simulink model "CLVF"  (R2020a)
settings: Solver=FixedStepAuto  StartTime=0.0  StopTime=tsim  FixedStep=baseRate  RelTol=1e-3  EnableMultiTasking=on
undefined symbols (not defined in the file): a, a_max, a_prime, acceptableRadius, b, baseRate, BLACKMass, d, DiscIntNeverNeededParam, Discrete, drop_states_BLACK, drop_states_BLUE, drop_states_RED, F_thrusters_BLACK, F_thrusters_BLUE, F_thrusters_RED, home_states_BLACK, home_states_BLUE, home_states_RED, init_states_BLACK, init_states_BLUE, init_states_RED, k_v_rel, ka, kc, kd, Kd_tb, Kd_tblue, Kd_tr, Kd_xb, Kd_xblue, Kd_xr, Kd_yb, Kd_yblue, Kd_yr, Kp_tb, Kp_tblue, Kp_tr, Kp_xb, Kp_xblue, Kp_xr, Kp_yb, Kp_yblue, Kp_yr, noise_variance_BLACK, noise_variance_BLUE, noise_variance_RED, o_hat_B, o_hat_prime, Phase0_End, Phase1_End, Phase2_End, Phase3_End, Phase3_SubPhase1_End, Phase3_SubPhase2_End, Phase3_SubPhase3_End, Phase3_SubPhase3_End_BLACK, Phase3_SubPhase3_End_RED, Phase3_SubPhase4_End, Phase4_End ... (+18)
libraries: dspsigops x14, dspstat3 x12, raspberrypiBasiclib x10, embdlinuxlib x8, simulink x8, ctrlSharedLib x4, mspfiltlib x3, dspswit3 x2, MainLibrary x2, dsparch4 x2, sensehatlib x1
(part 3 of 8)

== system CLVF/Phase #4: Return Home/Change RED Behavior ==
  note: ARM Control Law - RED
  note: PD Control Law - RED
  note: Additional Blocks
  note: Additional blocks are stored above. Note that to control attitude using the RW, simply replace RED_Tz with RED_Tz_RW.
  note: A simple PD control law is used here to command the platform to it's initial position, as defined in the initializer.
  note: This section is reserved for any control law for the robotic manipulator.
  Action Port : ActionPort  ActionPortLabel=if(u1 == 1 | u2 == 1)
  Constant : Constant  Value=home_states_RED(3)
  Constant1 : Constant  Value=home_states_RED(1)
  Constant{2,4..6} (4 alike) : Constant  Value=0
  Constant3 : Constant  Value=home_states_RED(2)
  Custom Discrete PD (Attitude) : Subsystem
  Custom Discrete PD (X-Position) : Subsystem
  Custom Discrete PD (Y-Position) : Subsystem
  Data Store Write : DataStoreWrite  DataStoreName=RED_Tz_Shoulder
  Data Store Write1 : DataStoreWrite  DataStoreName=RED_Tz_Elbow
  Data Store Write2 : DataStoreWrite  DataStoreName=RED_Tz_Wrist
  Data Store Write3 : DataStoreWrite  DataStoreName=Float_State
  Hough Control : Subsystem
  Puck State : Constant
  RED_Fx : DataStoreWrite  DataStoreName=RED_Fx
  RED_Fy : DataStoreWrite  DataStoreName=RED_Fy
  RED_Px : DataStoreRead  DataStoreName=RED_Px
  "RED_Py " : DataStoreRead  DataStoreName=RED_Py
  RED_Rz : DataStoreRead  DataStoreName=RED_Rz
  RED_Tz : DataStoreWrite  DataStoreName=RED_Tz
  RED_Tz_RW1 : DataStoreWrite  DataStoreName=RED_Tz_RW
  Subtract : Sum  Inputs=+-
  Subtract1 : Sum  Inputs=+-
  wires:
  Constant6/1 -> Data Store Write2/1
  Constant5/1 -> Data Store Write1/1
  Constant2/1 -> RED_Tz_RW1/1
  Constant4/1 -> Data Store Write/1
  Constant1/1 -> Subtract/1
  Custom Discrete PD (Attitude)/1(Tz) -> RED_Tz/1
  Constant/1 -> Hough Control/1(Ref)
  RED_Rz/1 -> Hough Control/2(Act)
  Constant3/1 -> Subtract1/1
  Custom Discrete PD (X-Position)/1(Fx) -> RED_Fx/1
  Subtract/1 -> Custom Discrete PD (X-Position)/1(ex)
  Hough Control/1(Err) -> Custom Discrete PD (Attitude)/1(ez)
  Custom Discrete PD (Y-Position)/1(Fy) -> RED_Fy/1
  RED_Px/1 -> Subtract/2
  "RED_Py "/1 -> Subtract1/2
  Subtract1/1 -> Custom Discrete PD (Y-Position)/1(ey)
  Puck State/1 -> Data Store Write3/1

== system CLVF/Phase #4: Return Home/Is this a simulation? ==
  Constant : Constant  Value=simMode  SampleTime=-1
  isSim : Outport  VectorParamsAs1DForOutWhenUnconnected=off
  wires:
  Constant/1 -> isSim/1

== system CLVF/Phase #5: Hold Home/Change BLACK Behavior ==
  note: Additional Blocks
  note: PD Control Law - BLACK
  note: A simple PD control law is used here to command the platform to it's initial position, as defined in the initializer.
  note: Additional blocks are stored here.
  Action Port : ActionPort  ActionPortLabel=if(u1 == 2 | u2 == 1)
  BLACK_Fx : DataStoreWrite  DataStoreName=BLACK_Fx
  BLACK_Fy : DataStoreWrite  DataStoreName=BLACK_Fy
  BLACK_Px : DataStoreRead  DataStoreName=BLACK_Px
  "BLACK_Py " : DataStoreRead  DataStoreName=BLACK_Py
  BLACK_Rz : DataStoreRead  DataStoreName=BLACK_Rz
  BLACK_Tz : DataStoreWrite  DataStoreName=BLACK_Tz
  Constant : Constant  Value=home_states_BLACK(1)
  Constant2 : Constant  Value=home_states_BLACK(2)
  Constant3 : Constant  Value=home_states_BLACK(3)
  Custom Discrete PD (Attitude) : Subsystem
  Custom Discrete PD (X-Position) : Subsystem
  Custom Discrete PD (Y-Position) : Subsystem
  Data Store Write3 : DataStoreWrite  DataStoreName=Float_State
  Hough Control : Subsystem
  Puck State : Constant
  Subtract : Sum  Inputs=+-
  Subtract1 : Sum  Inputs=+-
  wires:
  Custom Discrete PD (X-Position)/1(Fx) -> BLACK_Fx/1
  "BLACK_Py "/1 -> Subtract1/2
  Subtract1/1 -> Custom Discrete PD (Y-Position)/1(ey)
  Custom Discrete PD (Y-Position)/1(Fy) -> BLACK_Fy/1
  Constant3/1 -> Hough Control/1(Ref)
  Constant/1 -> Subtract/1
  Constant2/1 -> Subtract1/1
  Subtract/1 -> Custom Discrete PD (X-Position)/1(ex)
  Hough Control/1(Err) -> Custom Discrete PD (Attitude)/1(ez)
  Custom Discrete PD (Attitude)/1(Tz) -> BLACK_Tz/1
  BLACK_Px/1 -> Subtract/2
  BLACK_Rz/1 -> Hough Control/2(Act)
  Puck State/1 -> Data Store Write3/1

== system CLVF/Phase #5: Hold Home/Change BLUE Behavior ==
  note: PD Control Law - WHITE
  note: Additional blocks are stored here.
  note: A simple PD control law is used here to command the platform to it's initial position, as defined in the initializer.
  note: Additional Blocks
  Action Port : ActionPort  ActionPortLabel=if(u1 == 3 | u2 == 1)
  BLUE_Fx : DataStoreWrite  DataStoreName=BLUE_Fx
  BLUE_Fy : DataStoreWrite  DataStoreName=BLUE_Fy
  BLUE_Px : DataStoreRead  DataStoreName=BLUE_Px
  "BLUE_Py " : DataStoreRead  DataStoreName=BLUE_Py
  BLUE_Rz : DataStoreRead  DataStoreName=BLUE_Rz
  BLUE_Tz : DataStoreWrite  DataStoreName=BLUE_Tz
  Custom Discrete PD (Attitude) : Subsystem
  Custom Discrete PD (X-Position) : Subsystem
  Custom Discrete PD (Y-Position) : Subsystem
  Data Store Write3 : DataStoreWrite  DataStoreName=Float_State
  Desired Attitude (BLUE) : Constant  Value=home_states_BLUE(3)  SampleTime=-1
  Desired Px (BLUE) : Constant  Value=home_states_BLUE(1)  SampleTime=-1
  Desired Py (BLUE) : Constant  Value=home_states_BLUE(2)  SampleTime=-1
  Hough Control : Subsystem
  Puck State : Constant
  Subtract : Sum  Inputs=+-
  Subtract1 : Sum  Inputs=+-
  wires:
  Puck State/1 -> Data Store Write3/1
  Custom Discrete PD (Y-Position)/1(Fy) -> BLUE_Fy/1
  Custom Discrete PD (X-Position)/1(Fx) -> BLUE_Fx/1
  Subtract1/1 -> Custom Discrete PD (Y-Position)/1(ey)
  "BLUE_Py "/1 -> Subtract1/2
  Desired Px (BLUE)/1 -> Subtract/1
  Hough Control/1(Err) -> Custom Discrete PD (Attitude)/1(ez)
  Subtract/1 -> Custom Discrete PD (X-Position)/1(ex)
  Custom Discrete PD (Attitude)/1(Tz) -> BLUE_Tz/1
  BLUE_Rz/1 -> Hough Control/2(Act)
  Desired Py (BLUE)/1 -> Subtract1/1
  BLUE_Px/1 -> Subtract/2
  Desired Attitude (BLUE)/1 -> Hough Control/1(Ref)

== system CLVF/Phase #5: Hold Home/Change RED Behavior ==
  note: PD Control Law - RED
  note: ARM Control Law - RED
  note: Additional Blocks
  note: Additional blocks are stored above. Note that to control attitude using the RW, simply replace RED_Tz with RED_Tz_RW.
  note: A simple PD control law is used here to command the platform to it's home position, as defined in the initializer.
  note: This section is reserved for any control law for the robotic manipulator.
  Action Port : ActionPort  ActionPortLabel=if(u1 == 1 | u2 == 1)
  Constant : Constant  Value=home_states_RED(1)
  Constant{1,4..6} (4 alike) : Constant  Value=0
  Constant2 : Constant  Value=home_states_RED(2)
  Constant3 : Constant  Value=home_states_RED(3)
  Custom Discrete PD (Attitude) : Subsystem
  Custom Discrete PD (X-Position) : Subsystem
  Custom Discrete PD (Y-Position) : Subsystem
  Data Store Write : DataStoreWrite  DataStoreName=RED_Tz_Shoulder
  Data Store Write1 : DataStoreWrite  DataStoreName=RED_Tz_Elbow
  Data Store Write2 : DataStoreWrite  DataStoreName=RED_Tz_Wrist
  Data Store Write3 : DataStoreWrite  DataStoreName=Float_State
  Hough Control : Subsystem
  Puck State : Constant
  RED_Fx : DataStoreWrite  DataStoreName=RED_Fx
  RED_Fy : DataStoreWrite  DataStoreName=RED_Fy
  RED_Px : DataStoreRead  DataStoreName=RED_Px
  "RED_Py " : DataStoreRead  DataStoreName=RED_Py
  RED_Rz : DataStoreRead  DataStoreName=RED_Rz
  RED_Tz : DataStoreWrite  DataStoreName=RED_Tz
  RED_Tz_RW : DataStoreWrite  DataStoreName=RED_Tz_RW
  Subtract : Sum  Inputs=+-
  Subtract1 : Sum  Inputs=+-
  wires:
  Constant1/1 -> RED_Tz_RW/1
  Constant5/1 -> Data Store Write1/1
  Constant4/1 -> Data Store Write/1
  Constant6/1 -> Data Store Write2/1
  "RED_Py "/1 -> Subtract1/2
  Custom Discrete PD (Attitude)/1(Tz) -> RED_Tz/1
  Subtract1/1 -> Custom Discrete PD (Y-Position)/1(ey)
  Hough Control/1(Err) -> Custom Discrete PD (Attitude)/1(ez)
  RED_Px/1 -> Subtract/2
  Custom Discrete PD (X-Position)/1(Fx) -> RED_Fx/1
  Subtract/1 -> Custom Discrete PD (X-Position)/1(ex)
  Custom Discrete PD (Y-Position)/1(Fy) -> RED_Fy/1
  Constant/1 -> Subtract/1
  Constant3/1 -> Hough Control/1(Ref)
  RED_Rz/1 -> Hough Control/2(Act)
  Constant2/1 -> Subtract1/1
  Puck State/1 -> Data Store Write3/1

== system CLVF/Phase #5: Hold Home/Is this a simulation? ==
  Constant : Constant  Value=simMode  SampleTime=-1
  isSim : Outport  VectorParamsAs1DForOutWhenUnconnected=off
  wires:
  Constant/1 -> isSim/1

== system CLVF/Phase #6: Stop Floating and Spin Down RW/Change BLACK Behavior ==
  note: At the end of the experiment, the pucks must be turned off.
  note: At the end of the experiment, all thrust and arms movement must cease.
  Action Port : ActionPort  ActionPortLabel=if(u1 == 2 | u2 == 1)
  BLACK_Fx : DataStoreWrite  DataStoreName=BLACK_Fx
  BLACK_Fy : DataStoreWrite  DataStoreName=BLACK_Fy
  BLACK_Tz : DataStoreWrite  DataStoreName=BLACK_Tz
  Constant3 : Constant  Value=0
  Constant4 : Constant  Value=0
  Constant5 : Constant  Value=0
  Data Store Write3 : DataStoreWrite  DataStoreName=Float_State
  Puck State : Constant  Value=0
  wires:
  Constant3/1 -> BLACK_Fx/1
  Constant5/1 -> BLACK_Tz/1
  Constant4/1 -> BLACK_Fy/1
  Puck State/1 -> Data Store Write3/1

== system CLVF/Phase #6: Stop Floating and Spin Down RW/Change BLUE Behavior ==
  note: Before getting good data, the platforms must NOT be floating. So, float is set to be "off".
  note: For the initialization phase, we do not want any thrust. Thus, all commanded forces are zero.
  Action Port : ActionPort  ActionPortLabel=if(u1 == 3 | u2 == 1)
  BLUE_Fx : DataStoreWrite  DataStoreName=BLUE_Fx
  BLUE_Fy : DataStoreWrite  DataStoreName=BLUE_Fy
  BLUE_Tz : DataStoreWrite  DataStoreName=BLUE_Tz
  Constant3 : Constant  Value=0
  Constant4 : Constant  Value=0
  Constant5 : Constant  Value=0
  Data Store Write4 : DataStoreWrite  DataStoreName=Float_State
  Puck State : Constant  Value=0
  wires:
  Constant3/1 -> BLUE_Fx/1
  Constant5/1 -> BLUE_Tz/1
  Constant4/1 -> BLUE_Fy/1
  Puck State/1 -> Data Store Write4/1

== system CLVF/Phase #6: Stop Floating and Spin Down RW/Change RED Behavior ==
  note: At the end of the experiment, the pucks must be turned off.
  note: At the end of the experiment, all thrust and arms movement must cease.
  note: Once the platform has settled, the RW must be slowly desaturated (assuming it has been used).
  Action Port : ActionPort  ActionPortLabel=if(u1 == 1 | u2 == 1)
  Constant{,1..2,4..6} (6 alike) : Constant  Value=0
  Data Store Write : DataStoreWrite  DataStoreName=RED_Tz_Shoulder
  Data Store Write1 : DataStoreWrite  DataStoreName=RED_Tz_Elbow
  Data Store Write2 : DataStoreWrite  DataStoreName=RED_Tz_Wrist
  Data Store Write3 : DataStoreWrite  DataStoreName=Float_State
  Gain : Gain  Gain=-1
  Puck State : Constant  Value=0
  RED_Fx : DataStoreWrite  DataStoreName=RED_Fx
  RED_Fy : DataStoreWrite  DataStoreName=RED_Fy
  RED_Tz : DataStoreWrite  DataStoreName=RED_Tz
  RED_Tz_RW : DataStoreWrite  DataStoreName=RED_Tz_RW
  RED_dRz_Speed : DataStoreRead  DataStoreName=RED_dRz_RW_Sat
  Saturation : Saturate  UpperLimit=0.005  LowerLimit=-0.005
  wires:
  Constant/1 -> RED_Fx/1
  Constant6/1 -> Data Store Write2/1
  Constant5/1 -> Data Store Write1/1
  RED_dRz_Speed/1 -> Gain/1
  Constant4/1 -> Data Store Write/1
  Saturation/1 -> RED_Tz_RW/1
  Constant1/1 -> RED_Fy/1
  Gain/1 -> Saturation/1
  Constant2/1 -> RED_Tz/1
  Puck State/1 -> Data Store Write3/1

== system CLVF/Phase #6: Stop Floating and Spin Down RW/Is this a simulation? ==
  Constant : Constant  Value=simMode  SampleTime=-1
  isSim : Outport  VectorParamsAs1DForOutWhenUnconnected=off
  wires:
  Constant/1 -> isSim/1

== system CLVF/Simulate Plant Dynamics/BLACK Dynamics Model ==
  control_inputs : Inport
  Acceleration to Velocity : DiscreteIntegrator  SampleTime=-1  ICPrevOutput=DiscIntNeverNeededParam  ICPrevScaledInput=DiscIntNeverNeededParam
  MATLAB Function : MATLAB Function  TreatAsAtomicUnit=on
  Random Number : RandomNumber  Variance=noise_variance_BLACK
  Sum : Sum  Inputs=|++
  Velocity to Position : DiscreteIntegrator  InitialCondition=drop_states_BLACK  SampleTime=-1  ICPrevOutput=DiscIntNeverNeededParam  ICPrevScaledInput=DiscIntNeverNeededParam
  states : Outport  VectorParamsAs1DForOutWhenUnconnected=off
  wires:
  control_inputs/1 -> MATLAB Function/1(control_inputs)
  MATLAB Function/1(x_ddot) -> Acceleration to Velocity/1
  Acceleration to Velocity/1 -> Velocity to Position/1
  Velocity to Position/1 -> Sum/1
  Sum/1 -> states/1
  Random Number/1 -> Sum/2

== system CLVF/Simulate Plant Dynamics/BLUE  Dynamics Model ==
  control_inputs : Inport
  Acceleration to Velocity : DiscreteIntegrator  SampleTime=-1  ICPrevOutput=DiscIntNeverNeededParam  ICPrevScaledInput=DiscIntNeverNeededParam
  MATLAB Function : MATLAB Function  TreatAsAtomicUnit=on
  Random Number : RandomNumber  Variance=noise_variance_BLUE
  Sum : Sum  Inputs=|++
  Velocity to Position : DiscreteIntegrator  InitialCondition=drop_states_BLUE  SampleTime=-1  ICPrevOutput=DiscIntNeverNeededParam  ICPrevScaledInput=DiscIntNeverNeededParam
  states : Outport  VectorParamsAs1DForOutWhenUnconnected=off
  wires:
  control_inputs/1 -> MATLAB Function/1(control_inputs)
  MATLAB Function/1(x_ddot) -> Acceleration to Velocity/1
  Acceleration to Velocity/1 -> Velocity to Position/1
  Velocity to Position/1 -> Sum/1
  Sum/1 -> states/1
  Random Number/1 -> Sum/2

== system CLVF/Simulate Plant Dynamics/RED Dynamics Model ==
  control_inputs : Inport
  Acceleration to Velocity : DiscreteIntegrator  SampleTime=-1  ICPrevOutput=DiscIntNeverNeededParam  ICPrevScaledInput=DiscIntNeverNeededParam
  MATLAB Function : MATLAB Function  TreatAsAtomicUnit=on
  Random Number : RandomNumber  Variance=noise_variance_RED
  Sum : Sum  Inputs=|++
  Velocity to Position : DiscreteIntegrator  InitialCondition=drop_states_RED  SampleTime=-1  ICPrevOutput=DiscIntNeverNeededParam  ICPrevScaledInput=DiscIntNeverNeededParam
  states : Outport  VectorParamsAs1DForOutWhenUnconnected=off
  wires:
  control_inputs/1 -> MATLAB Function/1(control_inputs)
  MATLAB Function/1(x_ddot) -> Acceleration to Velocity/1
  Acceleration to Velocity/1 -> Velocity to Position/1
  Velocity to Position/1 -> Sum/1
  Sum/1 -> states/1
  Random Number/1 -> Sum/2

== system CLVF/Simulate Plant Dynamics/Sample and Hold Data to Match PhaseSpace (BLACK) ==
  states : Inport
  Constant1 : Constant  Value=serverRate
  Data Store Read2 : DataStoreRead  DataStoreName=Univ_Time
  MATLAB Function : MATLAB Function  TreatAsAtomicUnit=on
  Sample and Hold1 : dspsigops/Sample and Hold  trig=Rising edge  initCond=drop_states_BLACK  latchinput=off
  states_hold : Outport  VectorParamsAs1DForOutWhenUnconnected=off
  wires:
  states/1 -> Sample and Hold1/1
  Data Store Read2/1 -> MATLAB Function/1(TIME)
  Constant1/1 -> MATLAB Function/2(SERVER)
  MATLAB Function/1(y) -> Sample and Hold1/Trigger
  Sample and Hold1/1 -> states_hold/1

== system CLVF/Simulate Plant Dynamics/Sample and Hold Data to Match PhaseSpace (BLUE) ==
  states : Inport
  Constant1 : Constant  Value=serverRate
  Data Store Read2 : DataStoreRead  DataStoreName=Univ_Time
  MATLAB Function : MATLAB Function  TreatAsAtomicUnit=on
  Sample and Hold1 : dspsigops/Sample and Hold  trig=Rising edge  initCond=drop_states_BLUE  latchinput=off
  states_hold : Outport  VectorParamsAs1DForOutWhenUnconnected=off
  wires:
  states/1 -> Sample and Hold1/1
  Data Store Read2/1 -> MATLAB Function/1(TIME)
  Constant1/1 -> MATLAB Function/2(SERVER)
  MATLAB Function/1(y) -> Sample and Hold1/Trigger
  Sample and Hold1/1 -> states_hold/1

== system CLVF/Simulate Plant Dynamics/Sample and Hold Data to Match PhaseSpace (RED) ==
  states : Inport
  Constant : Constant  Value=serverRate
  Data Store Read1 : DataStoreRead  DataStoreName=Univ_Time
  MATLAB Function : MATLAB Function  TreatAsAtomicUnit=on
  Sample and Hold : dspsigops/Sample and Hold  trig=Rising edge  initCond=drop_states_RED  latchinput=off
  "states_hold " : Outport  VectorParamsAs1DForOutWhenUnconnected=off
  wires:
  Data Store Read1/1 -> MATLAB Function/1(TIME)
  Constant/1 -> MATLAB Function/2(SERVER)
  MATLAB Function/1(y) -> Sample and Hold/Trigger
  Sample and Hold/1 -> "states_hold "/1
  states/1 -> Sample and Hold/1

== system CLVF/Simulate Plant Dynamics/x_dot -> x1 ==
  note: dy/dt ~= (y2-y1)/deltaT
  y(t) : Inport
  Delay1 : Delay  DelayLength=1  InitialConditionSource=Input port
      settings: InputPortMap=u0,p4
  Hold this value : Subsystem  TreatAsAtomicUnit=on
  Sum6 : Sum  Inputs=-+|
  divide by delta T : Gain  Gain=1/serverRate
  "if we went through a \"step\"" : If  IfExpression=u1 ~= 0  ShowElse=off
  dy(t)/dt : Outport  VectorParamsAs1DForOutWhenUnconnected=off
  wires:
  divide by delta T/1 -> dy(t)/dt/1
  Delay1/1 -> Sum6/1
  "if we went through a \"step\""/1 -> Hold this value/Action
  Hold this value/1(Out1) -> divide by delta T/1
  Sum6/1 -> "if we went through a \"step\""/1, Hold this value/1(In1)
  y(t)/1 -> Sum6/2, Delay1/2, Delay1/1

== system CLVF/Simulate Plant Dynamics/x_dot -> x10 ==
  note: dy/dt ~= (y2-y1)/deltaT
  y(t) : Inport
  Delay1 : Delay  DelayLength=1  InitialConditionSource=Input port
      settings: InputPortMap=u0,p4
  Hold this value : Subsystem  TreatAsAtomicUnit=on
  Sum6 : Sum  Inputs=-+|
  divide by delta T : Gain  Gain=1/serverRate
  "if we went through a \"step\"" : If  IfExpression=u1 ~= 0  ShowElse=off
  dy(t)/dt : Outport  VectorParamsAs1DForOutWhenUnconnected=off
  wires:
  divide by delta T/1 -> dy(t)/dt/1
  Delay1/1 -> Sum6/1
  "if we went through a \"step\""/1 -> Hold this value/Action
  Hold this value/1(Out1) -> divide by delta T/1
  Sum6/1 -> "if we went through a \"step\""/1, Hold this value/1(In1)
  y(t)/1 -> Sum6/2, Delay1/2, Delay1/1

== system CLVF/Simulate Plant Dynamics/x_dot -> x11 ==
  note: dy/dt ~= (y2-y1)/deltaT
  y(t) : Inport
  Delay1 : Delay  DelayLength=1  InitialConditionSource=Input port
      settings: InputPortMap=u0,p4
  Hold this value : Subsystem  TreatAsAtomicUnit=on
  Sum6 : Sum  Inputs=-+|
  divide by delta T : Gain  Gain=1/serverRate
  "if we went through a \"step\"" : If  IfExpression=u1 ~= 0  ShowElse=off
  dy(t)/dt : Outport  VectorParamsAs1DForOutWhenUnconnected=off
  wires:
  divide by delta T/1 -> dy(t)/dt/1
  Delay1/1 -> Sum6/1
  "if we went through a \"step\""/1 -> Hold this value/Action
  Hold this value/1(Out1) -> divide by delta T/1
  Sum6/1 -> "if we went through a \"step\""/1, Hold this value/1(In1)
  y(t)/1 -> Sum6/2, Delay1/2, Delay1/1

== system CLVF/Simulate Plant Dynamics/x_dot -> x13 ==
  note: dy/dt ~= (y2-y1)/deltaT
  y(t) : Inport
  Delay1 : Delay  DelayLength=1  InitialConditionSource=Input port
      settings: InputPortMap=u0,p4
  Hold this value : Subsystem  TreatAsAtomicUnit=on
  Sum6 : Sum  Inputs=-+|
  divide by delta T : Gain  Gain=1/serverRate
  "if we went through a \"step\"" : If  IfExpression=u1 ~= 0  ShowElse=off
  dy(t)/dt : Outport  VectorParamsAs1DForOutWhenUnconnected=off
  wires:
  divide by delta T/1 -> dy(t)/dt/1
  Delay1/1 -> Sum6/1
  "if we went through a \"step\""/1 -> Hold this value/Action
  Hold this value/1(Out1) -> divide by delta T/1
  Sum6/1 -> "if we went through a \"step\""/1, Hold this value/1(In1)
  y(t)/1 -> Sum6/2, Delay1/2, Delay1/1

== system CLVF/Simulate Plant Dynamics/x_dot -> x14 ==
  note: dy/dt ~= (y2-y1)/deltaT
  y(t) : Inport
  Delay1 : Delay  DelayLength=1  InitialConditionSource=Input port
      settings: InputPortMap=u0,p4
  Hold this value : Subsystem  TreatAsAtomicUnit=on
  Sum6 : Sum  Inputs=-+|
  divide by delta T : Gain  Gain=1/serverRate
  "if we went through a \"step\"" : If  IfExpression=u1 ~= 0  ShowElse=off
  dy(t)/dt : Outport  VectorParamsAs1DForOutWhenUnconnected=off
  wires:
  divide by delta T/1 -> dy(t)/dt/1
  Delay1/1 -> Sum6/1
  "if we went through a \"step\""/1 -> Hold this value/Action
  Hold this value/1(Out1) -> divide by delta T/1
  Sum6/1 -> "if we went through a \"step\""/1, Hold this value/1(In1)
  y(t)/1 -> Sum6/2, Delay1/2, Delay1/1

== system CLVF/Simulate Plant Dynamics/x_dot -> x16 ==
  note: dy/dt ~= (y2-y1)/deltaT
  y(t) : Inport
  Delay1 : Delay  DelayLength=1  InitialConditionSource=Input port
      settings: InputPortMap=u0,p4
  Hold this value : Subsystem  TreatAsAtomicUnit=on
  Sum6 : Sum  Inputs=-+|
  divide by delta T : Gain  Gain=1/serverRate
  "if we went through a \"step\"" : If  IfExpression=u1 ~= 0  ShowElse=off
  dy(t)/dt : Outport  VectorParamsAs1DForOutWhenUnconnected=off
  wires:
  divide by delta T/1 -> dy(t)/dt/1
  Delay1/1 -> Sum6/1
  "if we went through a \"step\""/1 -> Hold this value/Action
  Hold this value/1(Out1) -> divide by delta T/1
  Sum6/1 -> "if we went through a \"step\""/1, Hold this value/1(In1)
  y(t)/1 -> Sum6/2, Delay1/2, Delay1/1

== system CLVF/Simulate Plant Dynamics/x_dot -> x17 ==
  note: dy/dt ~= (y2-y1)/deltaT
  y(t) : Inport
  Delay1 : Delay  DelayLength=1  InitialConditionSource=Input port
      settings: InputPortMap=u0,p4
  Hold this value : Subsystem  TreatAsAtomicUnit=on
  Sum6 : Sum  Inputs=-+|
  divide by delta T : Gain  Gain=1/serverRate
  "if we went through a \"step\"" : If  IfExpression=u1 ~= 0  ShowElse=off
  dy(t)/dt : Outport  VectorParamsAs1DForOutWhenUnconnected=off
  wires:
  divide by delta T/1 -> dy(t)/dt/1
  Delay1/1 -> Sum6/1
  "if we went through a \"step\""/1 -> Hold this value/Action
  Hold this value/1(Out1) -> divide by delta T/1
  Sum6/1 -> "if we went through a \"step\""/1, Hold this value/1(In1)
  y(t)/1 -> Sum6/2, Delay1/2, Delay1/1

== system CLVF/Simulate Plant Dynamics/x_dot -> x2 ==
  note: dy/dt ~= (y2-y1)/deltaT
  y(t) : Inport
  Delay1 : Delay  DelayLength=1  InitialConditionSource=Input port
      settings: InputPortMap=u0,p4
  Hold this value : Subsystem  TreatAsAtomicUnit=on
  Sum6 : Sum  Inputs=-+|
  divide by delta T : Gain  Gain=1/serverRate
  "if we went through a \"step\"" : If  IfExpression=u1 ~= 0  ShowElse=off
  dy(t)/dt : Outport  VectorParamsAs1DForOutWhenUnconnected=off
  wires:
  divide by delta T/1 -> dy(t)/dt/1
  Delay1/1 -> Sum6/1
  "if we went through a \"step\""/1 -> Hold this value/Action
  Hold this value/1(Out1) -> divide by delta T/1
  Sum6/1 -> "if we went through a \"step\""/1, Hold this value/1(In1)
  y(t)/1 -> Sum6/2, Delay1/2, Delay1/1

== system CLVF/Simulate Plant Dynamics/x_dot -> x3 ==
  note: dy/dt ~= (y2-y1)/deltaT
  y(t) : Inport
  Delay1 : Delay  DelayLength=1  InitialConditionSource=Input port
      settings: InputPortMap=u0,p4
  Hold this value : Subsystem  TreatAsAtomicUnit=on
  Sum6 : Sum  Inputs=-+|
  divide by delta T : Gain  Gain=1/serverRate
  "if we went through a \"step\"" : If  IfExpression=u1 ~= 0  ShowElse=off
  dy(t)/dt : Outport  VectorParamsAs1DForOutWhenUnconnected=off
  wires:
  divide by delta T/1 -> dy(t)/dt/1
  Delay1/1 -> Sum6/1
  "if we went through a \"step\""/1 -> Hold this value/Action
  Hold this value/1(Out1) -> divide by delta T/1
  Sum6/1 -> "if we went through a \"step\""/1, Hold this value/1(In1)
  y(t)/1 -> Sum6/2, Delay1/2, Delay1/1

== system CLVF/Simulate Plant Dynamics/x_dot -> x4 ==
  note: dy/dt ~= (y2-y1)/deltaT
  y(t) : Inport
  Delay1 : Delay  DelayLength=1  InitialConditionSource=Input port
      settings: InputPortMap=u0,p4
  Hold this value : Subsystem  TreatAsAtomicUnit=on
  Sum6 : Sum  Inputs=-+|
  divide by delta T : Gain  Gain=1/serverRate
  "if we went through a \"step\"" : If  IfExpression=u1 ~= 0  ShowElse=off
  dy(t)/dt : Outport  VectorParamsAs1DForOutWhenUnconnected=off
  wires:
  divide by delta T/1 -> dy(t)/dt/1
  Delay1/1 -> Sum6/1
  "if we went through a \"step\""/1 -> Hold this value/Action
  Hold this value/1(Out1) -> divide by delta T/1
  Sum6/1 -> "if we went through a \"step\""/1, Hold this value/1(In1)
  y(t)/1 -> Sum6/2, Delay1/2, Delay1/1

== system CLVF/Simulate Plant Dynamics/x_dot -> x5 ==
  note: dy/dt ~= (y2-y1)/deltaT
  y(t) : Inport
  Delay1 : Delay  DelayLength=1  InitialConditionSource=Input port
      settings: InputPortMap=u0,p4
  Hold this value : Subsystem  TreatAsAtomicUnit=on
  Sum6 : Sum  Inputs=-+|
  divide by delta T : Gain  Gain=1/serverRate
  "if we went through a \"step\"" : If  IfExpression=u1 ~= 0  ShowElse=off
  dy(t)/dt : Outport  VectorParamsAs1DForOutWhenUnconnected=off
  wires:
  divide by delta T/1 -> dy(t)/dt/1
  Delay1/1 -> Sum6/1
  "if we went through a \"step\""/1 -> Hold this value/Action
  Hold this value/1(Out1) -> divide by delta T/1
  Sum6/1 -> "if we went through a \"step\""/1, Hold this value/1(In1)
  y(t)/1 -> Sum6/2, Delay1/2, Delay1/1

== system CLVF/Simulate Plant Dynamics/x_dot -> x6 ==
  note: dy/dt ~= (y2-y1)/deltaT
  y(t) : Inport
  Delay1 : Delay  DelayLength=1  InitialConditionSource=Input port
      settings: InputPortMap=u0,p4
  Hold this value : Subsystem  TreatAsAtomicUnit=on
  Sum6 : Sum  Inputs=-+|
  divide by delta T : Gain  Gain=1/serverRate
  "if we went through a \"step\"" : If  IfExpression=u1 ~= 0  ShowElse=off
  dy(t)/dt : Outport  VectorParamsAs1DForOutWhenUnconnected=off
  wires:
  divide by delta T/1 -> dy(t)/dt/1
  Delay1/1 -> Sum6/1
  "if we went through a \"step\""/1 -> Hold this value/Action
  Hold this value/1(Out1) -> divide by delta T/1
  Sum6/1 -> "if we went through a \"step\""/1, Hold this value/1(In1)
  y(t)/1 -> Sum6/2, Delay1/2, Delay1/1

== system CLVF/Simulate Plant Dynamics/x_dot -> x7 ==
  note: dy/dt ~= (y2-y1)/deltaT
  y(t) : Inport
  Delay1 : Delay  DelayLength=1  InitialConditionSource=Input port
      settings: InputPortMap=u0,p4
  Hold this value : Subsystem  TreatAsAtomicUnit=on
  Sum6 : Sum  Inputs=-+|
  divide by delta T : Gain  Gain=1/serverRate
  "if we went through a \"step\"" : If  IfExpression=u1 ~= 0  ShowElse=off
  dy(t)/dt : Outport  VectorParamsAs1DForOutWhenUnconnected=off
  wires:
  divide by delta T/1 -> dy(t)/dt/1
  Delay1/1 -> Sum6/1
  "if we went through a \"step\""/1 -> Hold this value/Action
  Hold this value/1(Out1) -> divide by delta T/1
  Sum6/1 -> "if we went through a \"step\""/1, Hold this value/1(In1)
  y(t)/1 -> Sum6/2, Delay1/2, Delay1/1

== system CLVF/Simulate Plant Dynamics/x_dot -> x8 ==
  note: dy/dt ~= (y2-y1)/deltaT
  y(t) : Inport
  Delay1 : Delay  DelayLength=1  InitialConditionSource=Input port
      settings: InputPortMap=u0,p4
  Hold this value : Subsystem  TreatAsAtomicUnit=on
  Sum6 : Sum  Inputs=-+|
  divide by delta T : Gain  Gain=1/serverRate
  "if we went through a \"step\"" : If  IfExpression=u1 ~= 0  ShowElse=off
  dy(t)/dt : Outport  VectorParamsAs1DForOutWhenUnconnected=off
  wires:
  divide by delta T/1 -> dy(t)/dt/1
  Delay1/1 -> Sum6/1
  "if we went through a \"step\""/1 -> Hold this value/Action
  Hold this value/1(Out1) -> divide by delta T/1
  Sum6/1 -> "if we went through a \"step\""/1, Hold this value/1(In1)
  y(t)/1 -> Sum6/2, Delay1/2, Delay1/1

== system CLVF/Simulate Plant Dynamics/x_dot -> x9 ==
  note: dy/dt ~= (y2-y1)/deltaT
  y(t) : Inport
  Delay1 : Delay  DelayLength=1  InitialConditionSource=Input port
      settings: InputPortMap=u0,p4
  Hold this value : Subsystem  TreatAsAtomicUnit=on
  Sum6 : Sum  Inputs=-+|
  divide by delta T : Gain  Gain=1/serverRate
  "if we went through a \"step\"" : If  IfExpression=u1 ~= 0  ShowElse=off
  dy(t)/dt : Outport  VectorParamsAs1DForOutWhenUnconnected=off
  wires:
  divide by delta T/1 -> dy(t)/dt/1
  Delay1/1 -> Sum6/1
  "if we went through a \"step\""/1 -> Hold this value/Action
  Hold this value/1(Out1) -> divide by delta T/1
  Sum6/1 -> "if we went through a \"step\""/1, Hold this value/1(In1)
  y(t)/1 -> Sum6/2, Delay1/2, Delay1/1

== system CLVF/From Force//Torque to PWM Signal/Change BLACK Behavior/Calculate Thruster ON//OFF ==
  note: Calculate which thrusters must be turned on and for how long.
  note: The H matrix is not square, thus a pserudo-inverse is required.
  note: Knowing how much force each thruster can output, we can determine the saturated thruster output and then convert is into a percentage of time over which each thruster is open.
  note: After finding the PWM value, we can use the H matrix to go back to torque and force. However, these torques and forces will be "saturated".
  "[Fx_b; Fy_b; Tz]" : Inport
  BLACK_Fx_Sat : DataStoreWrite  DataStoreName=BLACK_Fx_Sat
  BLACK_Fy_Sat : DataStoreWrite  DataStoreName=BLACK_Fy_Sat
  BLACK_Rz : DataStoreRead  DataStoreName=BLACK_Rz
  BLACK_Tz_Sat : DataStoreWrite  DataStoreName=BLACK_Tz_Sat
  Demux : Demux  Outputs=3
  Demux1 : Demux  Outputs=2
  MATLAB Function : MATLAB Function  TreatAsAtomicUnit=on
  MATLAB Function1 : MATLAB Function  TreatAsAtomicUnit=on
  MATLAB Function2 : MATLAB Function  TreatAsAtomicUnit=on
  Mux : Mux  Inputs=2
  Product : Product  Multiplication=Matrix(*)
  Product1 : Product  Multiplication=Matrix(*)
  Remove Negatives : Saturate  UpperLimit=1000  LowerLimit=0
  Rotate Forces to Inertial : Subsystem
  pseudo-inverse : Subsystem
  ThrusterPWM : Outport  VectorParamsAs1DForOutWhenUnconnected=off
  wires:
  pseudo-inverse/1(invH) -> Product/1
  Product/1 -> Remove Negatives/1
  "[Fx_b; Fy_b; Tz]"/1 -> Product/2
  MATLAB Function/1(H) -> pseudo-inverse/1(H)
  Remove Negatives/1 -> MATLAB Function2/1(ThrustPer)
  MATLAB Function1/1(H) -> Product1/1
  Product1/1 -> Demux/1
  Demux/2 -> Mux/2
  Demux/1 -> Mux/1
  Mux/1 -> Rotate Forces to Inertial/1("F_b ")
  BLACK_Rz/1 -> Rotate Forces to Inertial/2(Rz)
  Demux/3 -> BLACK_Tz_Sat/1
  Rotate Forces to Inertial/1(F_I) -> Demux1/1
  Demux1/1 -> BLACK_Fx_Sat/1
  Demux1/2 -> BLACK_Fy_Sat/1
  MATLAB Function2/1(ThrustPer_Final) -> Product1/2, ThrusterPWM/1

== system CLVF/From Force//Torque to PWM Signal/Change BLACK Behavior/Rotate Forces to Body ==
  "F_I " : Inport
  Rz : Inport  Port=2
  Create Rotation Matrix : MATLAB Function  TreatAsAtomicUnit=on
  Rotate F_I to F_b : Product  Multiplication=Matrix(*)
  F_b : Outport  VectorParamsAs1DForOutWhenUnconnected=off
  wires:
  Rotate F_I to F_b/1 -> F_b/1
  Create Rotation Matrix/1(C_bI) -> Rotate F_I to F_b/1
  "F_I "/1 -> Rotate F_I to F_b/2
  Rz/1 -> Create Rotation Matrix/1(Rz)

== system CLVF/From Force//Torque to PWM Signal/Change BLUE Behavior/Calculate Thruster ON//OFF ==
  note: Calculate which thrusters must be turned on and for how long.
  note: The H matrix is not square, thus a pserudo-inverse is required.
  note: Knowing how much force each thruster can output, we can determine the saturated thruster output and then convert is into a percentage of time over which each thruster is open.
  note: After finding the PWM value, we can use the H matrix to go back to torque and force. However, these torques and forces will be "saturated".
  "[Fx_b; Fy_b; Tz]" : Inport
  BLUE_Fx_Sat : DataStoreWrite  DataStoreName=BLUE_Fx_Sat
  BLUE_Fy_Sat : DataStoreWrite  DataStoreName=BLUE_Fy_Sat
  BLUE_Rz : DataStoreRead  DataStoreName=BLUE_Rz
  BLUE_Tz_Sat : DataStoreWrite  DataStoreName=BLUE_Tz_Sat
  Demux : Demux  Outputs=3
  Demux1 : Demux  Outputs=2
  MATLAB Function : MATLAB Function  TreatAsAtomicUnit=on
  MATLAB Function1 : MATLAB Function  TreatAsAtomicUnit=on
  MATLAB Function2 : MATLAB Function  TreatAsAtomicUnit=on
  Mux : Mux  Inputs=2
  Product : Product  Multiplication=Matrix(*)
  Product1 : Product  Multiplication=Matrix(*)
  Remove Negatives : Saturate  UpperLimit=1000  LowerLimit=0
  Rotate Forces to Inertial : Subsystem
  pseudo-inverse : Subsystem
  ThrusterPWM : Outport  VectorParamsAs1DForOutWhenUnconnected=off
  wires:
  pseudo-inverse/1(invH) -> Product/1
  Product/1 -> Remove Negatives/1
  "[Fx_b; Fy_b; Tz]"/1 -> Product/2
  MATLAB Function/1(H) -> pseudo-inverse/1(H)
  Remove Negatives/1 -> MATLAB Function2/1(ThrustPer)
  MATLAB Function1/1(H) -> Product1/1
  Product1/1 -> Demux/1
  Demux/2 -> Mux/2
  Demux/1 -> Mux/1
  Mux/1 -> Rotate Forces to Inertial/1("F_b ")
  BLUE_Rz/1 -> Rotate Forces to Inertial/2(Rz)
  Demux/3 -> BLUE_Tz_Sat/1
  Rotate Forces to Inertial/1(F_I) -> Demux1/1
  Demux1/1 -> BLUE_Fx_Sat/1
  Demux1/2 -> BLUE_Fy_Sat/1
  MATLAB Function2/1(ThrustPer_Final) -> Product1/2, ThrusterPWM/1

== system CLVF/From Force//Torque to PWM Signal/Change BLUE Behavior/Rotate Forces to Body ==
  "F_I " : Inport
  Rz : Inport  Port=2
  Create Rotation Matrix : MATLAB Function  TreatAsAtomicUnit=on
  Rotate F_I to F_b : Product  Multiplication=Matrix(*)
  F_b : Outport  VectorParamsAs1DForOutWhenUnconnected=off
  wires:
  Rotate F_I to F_b/1 -> F_b/1
  Create Rotation Matrix/1(C_bI) -> Rotate F_I to F_b/1
  "F_I "/1 -> Rotate F_I to F_b/2
  Rz/1 -> Create Rotation Matrix/1(Rz)

== system CLVF/From Force//Torque to PWM Signal/Change RED Behavior/Calculate Thruster ON//OFF ==
  note: Calculate which thrusters must be turned on and for how long.
  note: The H matrix is not square, thus a pserudo-inverse is required.
  note: Knowing how much force each thruster can output, we can determine the saturated thruster output and then convert is into a percentage of time over which each thruster is open.
  note: After finding the PWM value, we can use the H matrix to go back to torque and force. However, these torques and forces will be "saturated".
  "[Fx_b; Fy_b; Tz]" : Inport
  Demux : Demux  Outputs=3
  Demux1 : Demux  Outputs=2
  MATLAB Function : MATLAB Function  TreatAsAtomicUnit=on
  MATLAB Function1 : MATLAB Function  TreatAsAtomicUnit=on
  MATLAB Function2 : MATLAB Function  TreatAsAtomicUnit=on
  Mux : Mux  Inputs=2
  Product : Product  Multiplication=Matrix(*)
  Product1 : Product  Multiplication=Matrix(*)
  RED_Fx_Sat : DataStoreWrite  DataStoreName=RED_Fx_Sat
  RED_Fy_Sat : DataStoreWrite  DataStoreName=RED_Fy_Sat
  RED_Rz : DataStoreRead  DataStoreName=RED_Rz
  RED_Tz_Sat : DataStoreWrite  DataStoreName=RED_Tz_Sat
  Remove Negatives : Saturate  UpperLimit=1000  LowerLimit=0
  Rotate Forces to Inertial : Subsystem
  pseudo-inverse : Subsystem
  ThrusterPWM : Outport  VectorParamsAs1DForOutWhenUnconnected=off
  wires:
  pseudo-inverse/1(invH) -> Product/1
  Product/1 -> Remove Negatives/1
  "[Fx_b; Fy_b; Tz]"/1 -> Product/2
  MATLAB Function/1(H) -> pseudo-inverse/1(H)
  Remove Negatives/1 -> MATLAB Function2/1(ThrustPer)
  MATLAB Function1/1(H) -> Product1/1
  Product1/1 -> Demux/1
  Demux/2 -> Mux/2
  Demux/1 -> Mux/1
  Mux/1 -> Rotate Forces to Inertial/1("F_b ")
  RED_Rz/1 -> Rotate Forces to Inertial/2(Rz)
  Demux/3 -> RED_Tz_Sat/1
  Rotate Forces to Inertial/1(F_I) -> Demux1/1
  Demux1/1 -> RED_Fx_Sat/1
  Demux1/2 -> RED_Fy_Sat/1
  MATLAB Function2/1(ThrustPer_Final) -> Product1/2, ThrusterPWM/1

== system CLVF/From Force//Torque to PWM Signal/Change RED Behavior/Rotate Forces to Body ==
  "F_I " : Inport
  Rz : Inport  Port=2
  Create Rotation Matrix : MATLAB Function  TreatAsAtomicUnit=on
  Rotate F_I to F_b : Product  Multiplication=Matrix(*)
  F_b : Outport  VectorParamsAs1DForOutWhenUnconnected=off
  wires:
  Rotate F_I to F_b/1 -> F_b/1
  Create Rotation Matrix/1(C_bI) -> Rotate F_I to F_b/1
  "F_I "/1 -> Rotate F_I to F_b/2
  Rz/1 -> Create Rotation Matrix/1(Rz)

== system CLVF/From Torque, Command RW/Change RED Behavior/Calculate Saturated RPM Signal ==
  Tz : Inport
  Calculate RW RPM Increment : MATLAB Function  TreatAsAtomicUnit=on
  Delay : Delay  DelayLength=1
  Saturate RPM : Saturate  UpperLimit=(7000*64/3375)  LowerLimit=-(7000*64/3375)
  Saturate Torque : Saturate  UpperLimit=0.1  LowerLimit=-0.1
  Sum : Sum  Inputs=|++
  RPM : Outport  VectorParamsAs1DForOutWhenUnconnected=off
  RPM_Sat : Outport  Port=2  VectorParamsAs1DForOutWhenUnconnected=off
  wires:
  Tz/1 -> Saturate Torque/1
  Saturate RPM/1 -> Delay/1
  Calculate RW RPM Increment/1(dRPM_RW) -> Sum/1
  Delay/1 -> Sum/2
  Sum/1 -> RPM/1, Saturate RPM/1
  Saturate Torque/1 -> RPM_Sat/1, Calculate RW RPM Increment/1(Tz_Sat)

== system CLVF/From Torque, Command RW/Change RED Behavior/Wheel RPM to PWM ==
  note: Check the GPIO pin to see if the RW is ready to receive a command.
  note: Convert the RPM to a PWM value.
  note: Indicate Motor direction (0 for CW and 1 for CCW)
  WheelRPM : Inport
  Abs : Abs
  Check if RW is Ready : MATLAB Function  TreatAsAtomicUnit=on
  Convert Wheel Rate to Motor Rate : Subsystem
  Delay Bank : Subsystem
  Get RW Direction : MATLAB Function  TreatAsAtomicUnit=on
  Obtain RW Status : Subsystem  TreatAsAtomicUnit=on
  RED_RW_Speed : DataStoreWrite  DataStoreName=RED_dRz_RW_Sat
  RPM to PWM Value : MATLAB Function  TreatAsAtomicUnit=on
  Saturate Motor : Saturate  UpperLimit=7000  LowerLimit=-7000
  Send Direction to Motor Controller : Subsystem  TreatAsAtomicUnit=on
  Send PWM to Motor Controller : Subsystem  TreatAsAtomicUnit=on
  Turn on Motor : Subsystem  TreatAsAtomicUnit=on
  wires:
  WheelRPM/1 -> Check if RW is Ready/2(WheelRPM_In)
  Convert Wheel Rate to Motor Rate/1(Motor RPM) -> Saturate Motor/1
  Check if RW is Ready/2(WheelRPM_Out) -> RED_RW_Speed/1, Convert Wheel Rate to Motor Rate/1(Wheel RPM)
  Saturate Motor/1 -> Abs/1, Get RW Direction/1(MotorRPM_Sat)
  Delay Bank/1(StatusVector) -> Check if RW is Ready/1(Status)
  Abs/1 -> RPM to PWM Value/1(MotorRPM_Sat)
  Get RW Direction/1(WheelDirection) -> Send Direction to Motor Controller/1(WheelDir)
  RPM to PWM Value/1(MotorPWM) -> Send PWM to Motor Controller/1(MotorPWM)
  Obtain RW Status/1(RW_Status) -> Delay Bank/1(Status)
  Check if RW is Ready/1(EnableSig) -> Turn on Motor/1(EnableSig)

== system CLVF/Grab PhaseSpace Data via UDP/Use Hardware to Obtain States/Using RED+BLACK, or RED+BLACK+ARM ==
  note: In this subsection, the "if" statements are used to determine two things: 1) whether or not a simulation is begin performed,
      | then 2) if an experiment is being performed, then which platform is the diagram compiled on. The "IdentifyPlatform" variable
      | is obtained from a text file location on each platform; each text file contains a unique identifier for each platform.
  Action Port : ActionPort  ActionPortLabel=elseif(u1 == 3| u1 == 4)
  Constant : Constant  Value=WhoAmI
  Is this a simulation? : Subsystem
  Obtain BLACK States : Subsystem  TreatAsAtomicUnit=on
  Obtain RED States : Subsystem  TreatAsAtomicUnit=on
  This IF block determines whether or not to run the BLACK sim/exp : If  NumInputs=2  IfExpression=u1 == 2 | u2 == 1  ShowElse=off
  "This IF block determines whether or not to run the RED sim/exp " : If  NumInputs=2  IfExpression=u1 == 1 | u2 == 1  ShowElse=off
  wires:
  "This IF block determines whether or not to run the RED sim/exp "/1 -> Obtain RED States/Action
  Constant/1 -> This IF block determines whether or not to run the BLACK sim/exp/1, "This IF block determines whether or not to run the RED sim/exp "/1
  Is this a simulation?/1(isSim) -> This IF block determines whether or not to run the BLACK sim/exp/2, "This IF block determines whether or not to run the RED sim/exp "/2
  This IF block determines whether or not to run the BLACK sim/exp/1 -> Obtain BLACK States/Action

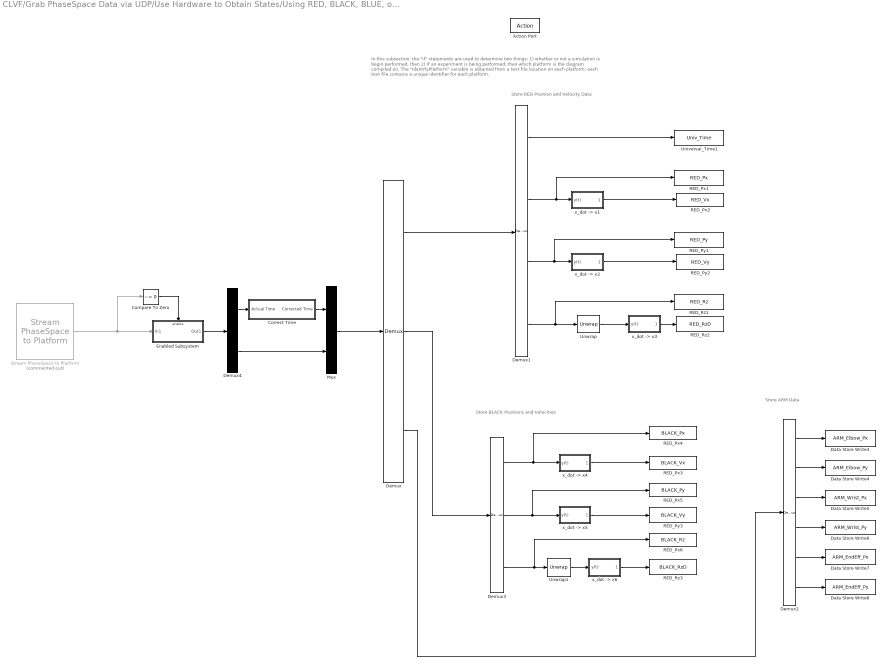
== system CLVF/Grab PhaseSpace Data via UDP/Use Hardware to Obtain States/Using RED, BLACK, BLUE, or RED + ARM ==
  note: In this subsection, the "if" statements are used to determine two things: 1) whether or not a simulation is begin performed,
      | then 2) if an experiment is being performed, then which platform is the diagram compiled on. The "IdentifyPlatform" variable
      | is obtained from a text file location on each platform; each text file contains a unique identifier for each platform.
  note: Store BLACK Positions and Velocities
  note: Store ARM Data
  note: Store RED Position and Velocity Data
  Action Port : ActionPort  ActionPortLabel=if(u1 == 1 | u1 == 2 | u1 == 5)
  Compare To Zero : simulink/Logic and Bit Operations/Compare To Zero  relop=~=  OutDataTypeStr=boolean
  Correct Time : Subsystem
  Data Store Write3 : DataStoreWrite  DataStoreName=ARM_Elbow_Px
  Data Store Write4 : DataStoreWrite  DataStoreName=ARM_Elbow_Py
  Data Store Write5 : DataStoreWrite  DataStoreName=ARM_Wrist_Px
  Data Store Write6 : DataStoreWrite  DataStoreName=ARM_Wrist_Py
  Data Store Write7 : DataStoreWrite  DataStoreName=ARM_EndEff_Px
  Data Store Write8 : DataStoreWrite  DataStoreName=ARM_EndEff_Py
  Demux : Demux  Outputs=[4,3,6]
  Demux1 : Demux
  Demux2 : Demux  Outputs=6
  Demux3 : Demux  Outputs=3
  Demux4 : Demux  Outputs=[1,12]
  Enabled Subsystem : Subsystem  TreatAsAtomicUnit=on
  Mux : Mux  Inputs=2
  RED_Px1 : DataStoreWrite  DataStoreName=RED_Px
  RED_Px2 : DataStoreWrite  DataStoreName=RED_Vx
  RED_Px3 : DataStoreWrite  DataStoreName=BLACK_Vx
  RED_Px4 : DataStoreWrite  DataStoreName=BLACK_Px
  RED_Px5 : DataStoreWrite  DataStoreName=BLACK_Py
  RED_Px6 : DataStoreWrite  DataStoreName=BLACK_Rz
  RED_Py1 : DataStoreWrite  DataStoreName=RED_Py
  RED_Py2 : DataStoreWrite  DataStoreName=RED_Vy
  RED_Py3 : DataStoreWrite  DataStoreName=BLACK_Vy
  RED_Rz1 : DataStoreWrite  DataStoreName=RED_Rz
  RED_Rz2 : DataStoreWrite  DataStoreName=RED_RzD
  RED_Rz3 : DataStoreWrite  DataStoreName=BLACK_RzD
  Stream PhaseSpace to Platform : MainLibrary/PhaseSpace Functions/Stream PhaseSpace to Platform  Commented=on  platformSelection=platformSelection
      settings: SourceProductName=SPOT Custom Library
  Universal_Time1 : DataStoreWrite  DataStoreName=Univ_Time
  Unwrap : dspsigops/Unwrap  tol=pi  InputProcessing=Columns as channels (frame based)  running=off
  Unwrap1 : dspsigops/Unwrap  tol=pi  InputProcessing=Columns as channels (frame based)  running=off
  "x_dot -> x1" : Subsystem
  "x_dot -> x2" : Subsystem
  "x_dot -> x3" : Subsystem
  "x_dot -> x4" : Subsystem
  "x_dot -> x5" : Subsystem
  "x_dot -> x6" : Subsystem
  wires:
  Demux3/1 -> "x_dot -> x4"/1(y(t)), RED_Px4/1
  Demux3/2 -> "x_dot -> x5"/1(y(t)), RED_Px5/1
  Demux1/3 -> "x_dot -> x2"/1(y(t)), RED_Py1/1
  Demux1/2 -> "x_dot -> x1"/1(y(t)), RED_Px1/1
  Demux3/3 -> Unwrap1/1, RED_Px6/1
  Demux2/5 -> Data Store Write7/1
  Demux2/2 -> Data Store Write4/1
  Demux1/1 -> Universal_Time1/1
  Demux4/1 -> Correct Time/1(Actual Time)
  Demux2/3 -> Data Store Write5/1
  Demux1/4 -> Unwrap/1, RED_Rz1/1
  "x_dot -> x5"/1(dy(t)/dt) -> RED_Py3/1
  Demux2/4 -> Data Store Write6/1
  "x_dot -> x4"/1(dy(t)/dt) -> RED_Px3/1
  Demux4/2 -> Mux/2
  Correct Time/1(Corrected Time) -> Mux/1
  "x_dot -> x1"/1(dy(t)/dt) -> RED_Px2/1
  Demux2/1 -> Data Store Write3/1
  Demux2/6 -> Data Store Write8/1
  Demux/2 -> Demux3/1
  Demux/1 -> Demux1/1
  "x_dot -> x2"/1(dy(t)/dt) -> RED_Py2/1
  "x_dot -> x6"/1(dy(t)/dt) -> RED_Rz3/1
  "x_dot -> x3"/1(dy(t)/dt) -> RED_Rz2/1
  Mux/1 -> Demux/1
  Unwrap/1 -> "x_dot -> x3"/1(y(t))
  Unwrap1/1 -> "x_dot -> x6"/1(y(t))
  Stream PhaseSpace to Platform/1 -> Enabled Subsystem/1(In1), Compare To Zero/1
  Enabled Subsystem/1(Out1) -> Demux4/1
  Compare To Zero/1 -> Enabled Subsystem/Enable
  Demux/3 -> Demux2/1

== system CLVF/Gyroscope & Acceleration Algorithms/Change BLACK Behavior/Fix Initial Bias ==
  Actual Gyro : Inport
  Correct GyroX : Subsystem
  Correct GyroY : Subsystem
  Correct GyroZ : Subsystem
  Demux : Demux  Outputs=3
  Mux : Mux  Inputs=3
  Corrected Gyro : Outport  VectorParamsAs1DForOutWhenUnconnected=off
  wires:
  Demux/1 -> Correct GyroX/1(In1)
  Demux/2 -> Correct GyroY/1(In1)
  Demux/3 -> Correct GyroZ/1(In1)
  Correct GyroX/1(Out1) -> Mux/1
  Correct GyroY/1(Out1) -> Mux/2
  Correct GyroZ/1(Out1) -> Mux/3
  Mux/1 -> Corrected Gyro/1
  Actual Gyro/1 -> Demux/1

== system CLVF/Gyroscope & Acceleration Algorithms/Change BLACK Behavior/Fix Initial Bias (Accel) ==
  Actual Accel : Inport
  Correct AccelX : Subsystem
  Correct AccelY : Subsystem
  Correct AccelZ : Subsystem
  Demux : Demux  Outputs=3
  Mux : Mux  Inputs=3
  Corrected Accel : Outport  VectorParamsAs1DForOutWhenUnconnected=off
  wires:
  Demux/1 -> Correct AccelX/1(In1)
  Demux/2 -> Correct AccelY/1(In1)
  Demux/3 -> Correct AccelZ/1(In1)
  Correct AccelX/1(Out1) -> Mux/1
  Correct AccelY/1(Out1) -> Mux/2
  Correct AccelZ/1(Out1) -> Mux/3
  Mux/1 -> Corrected Accel/1
  Actual Accel/1 -> Demux/1

== system CLVF/Gyroscope & Acceleration Algorithms/Change RED Behavior/Fix Initial Bias ==
  Actual Gyro : Inport
  Correct GyroX : Subsystem
  Correct GyroY : Subsystem
  Correct GyroZ : Subsystem
  Demux : Demux  Outputs=3
  Mux : Mux  Inputs=3
  Corrected Gyro : Outport  VectorParamsAs1DForOutWhenUnconnected=off
  wires:
  Demux/1 -> Correct GyroX/1(In1)
  Demux/2 -> Correct GyroY/1(In1)
  Demux/3 -> Correct GyroZ/1(In1)
  Correct GyroX/1(Out1) -> Mux/1
  Correct GyroY/1(Out1) -> Mux/2
  Correct GyroZ/1(Out1) -> Mux/3
  Mux/1 -> Corrected Gyro/1
  Actual Gyro/1 -> Demux/1

== system CLVF/Gyroscope & Acceleration Algorithms/Change RED Behavior/Fix Initial Bias (Accel) ==
  Actual Accel : Inport
  Correct AccelX : Subsystem
  Correct AccelY : Subsystem
  Correct AccelZ : Subsystem
  Demux : Demux  Outputs=3
  Mux : Mux  Inputs=3
  Corrected Accel : Outport  VectorParamsAs1DForOutWhenUnconnected=off
  wires:
  Demux/1 -> Correct AccelX/1(In1)
  Demux/2 -> Correct AccelY/1(In1)
  Demux/3 -> Correct AccelZ/1(In1)
  Correct AccelX/1(Out1) -> Mux/1
  Correct AccelY/1(Out1) -> Mux/2
  Correct AccelZ/1(Out1) -> Mux/3
  Mux/1 -> Corrected Accel/1
  Actual Accel/1 -> Demux/1

== system CLVF/Phase #2: Move to Initial Position/Change BLACK Behavior/Custom Discrete PD (Attitude) ==
  ez : Inport
  Sum3 : Sum
  kd_tb : Gain  Gain=Kd_tb
  kp_tb : Gain  Gain=Kp_tb
  "x_dot -> x1" : Subsystem
  Tz : Outport  VectorParamsAs1DForOutWhenUnconnected=off
  wires:
  kd_tb/1 -> Sum3/1
  Sum3/1 -> Tz/1
  kp_tb/1 -> Sum3/2
  "x_dot -> x1"/1(dy(t)/dt) -> kd_tb/1
  ez/1 -> "x_dot -> x1"/1(y(t)), kp_tb/1

== system CLVF/Phase #2: Move to Initial Position/Change BLACK Behavior/Custom Discrete PD (X-Position) ==
  ex : Inport
  Sum3 : Sum
  kd_xb : Gain  Gain=Kd_xb
  kp_xb : Gain  Gain=Kp_xb
  "x_dot -> x1" : Subsystem
  Fx : Outport  VectorParamsAs1DForOutWhenUnconnected=off
  wires:
  kd_xb/1 -> Sum3/1
  ex/1 -> "x_dot -> x1"/1(y(t)), kp_xb/1
  kp_xb/1 -> Sum3/2
  "x_dot -> x1"/1(dy(t)/dt) -> kd_xb/1
  Sum3/1 -> Fx/1

== system CLVF/Phase #2: Move to Initial Position/Change BLACK Behavior/Custom Discrete PD (Y-Position) ==
  ey : Inport
  Sum3 : Sum
  kd_yb : Gain  Gain=Kd_yb
  kp_yb : Gain  Gain=Kp_yb
  "x_dot -> x1" : Subsystem
  Fy : Outport  VectorParamsAs1DForOutWhenUnconnected=off
  wires:
  kd_yb/1 -> Sum3/1
  Sum3/1 -> Fy/1
  kp_yb/1 -> Sum3/2
  "x_dot -> x1"/1(dy(t)/dt) -> kd_yb/1
  ey/1 -> "x_dot -> x1"/1(y(t)), kp_yb/1

== system CLVF/Phase #2: Move to Initial Position/Change BLACK Behavior/Hough Control ==
  Ref : Inport
  Act : Inport  Port=2
  MATLAB Function2 : MATLAB Function  TreatAsAtomicUnit=on
  MATLAB Function3 : MATLAB Function  TreatAsAtomicUnit=on
  MATLAB Function4 : MATLAB Function  TreatAsAtomicUnit=on
  Subtract2 : Sum  Inputs=+-
  Err : Outport  VectorParamsAs1DForOutWhenUnconnected=off
  wires:
  MATLAB Function4/1(e_out) -> Err/1
  MATLAB Function2/1(Oy) -> MATLAB Function4/1(Oy)
  Subtract2/1 -> MATLAB Function4/2(e_in)
  MATLAB Function2/2(Ox) -> Subtract2/1
  Act/1 -> MATLAB Function3/1(z)
  Ref/1 -> MATLAB Function2/1(z)
  MATLAB Function3/1(Ox) -> Subtract2/2

== system CLVF/Phase #2: Move to Initial Position/Change BLUE Behavior/Custom Discrete PD (Attitude) ==
  ez : Inport
  Sum3 : Sum
  kd_tb : Gain  Gain=Kd_tblue
  kp_tb : Gain  Gain=Kp_tblue
  "x_dot -> x1" : Subsystem
  Tz : Outport  VectorParamsAs1DForOutWhenUnconnected=off
  wires:
  kd_tb/1 -> Sum3/1
  Sum3/1 -> Tz/1
  kp_tb/1 -> Sum3/2
  "x_dot -> x1"/1(dy(t)/dt) -> kd_tb/1
  ez/1 -> "x_dot -> x1"/1(y(t)), kp_tb/1

== system CLVF/Phase #2: Move to Initial Position/Change BLUE Behavior/Custom Discrete PD (X-Position) ==
  ex : Inport
  Sum3 : Sum
  kd_xb : Gain  Gain=Kd_xblue
  kp_xb : Gain  Gain=Kp_xblue
  "x_dot -> x1" : Subsystem
  Fx : Outport  VectorParamsAs1DForOutWhenUnconnected=off
  wires:
  kd_xb/1 -> Sum3/1
  ex/1 -> "x_dot -> x1"/1(y(t)), kp_xb/1
  kp_xb/1 -> Sum3/2
  "x_dot -> x1"/1(dy(t)/dt) -> kd_xb/1
  Sum3/1 -> Fx/1

== system CLVF/Phase #2: Move to Initial Position/Change BLUE Behavior/Custom Discrete PD (Y-Position) ==
  ey : Inport
  Sum3 : Sum
  kd_yb : Gain  Gain=Kd_yblue
  kp_yb : Gain  Gain=Kp_yblue
  "x_dot -> x1" : Subsystem
  Fy : Outport  VectorParamsAs1DForOutWhenUnconnected=off
  wires:
  kd_yb/1 -> Sum3/1
  Sum3/1 -> Fy/1
  kp_yb/1 -> Sum3/2
  "x_dot -> x1"/1(dy(t)/dt) -> kd_yb/1
  ey/1 -> "x_dot -> x1"/1(y(t)), kp_yb/1
